simulink model "tank2_update"  (R2014a)
settings: Solver=ode1  StartTime=0.0  StopTime=inf  FixedStep=delta_t  RelTol=1e-3
PreLoadFcn:
  | model_prediction_init
undefined symbols (not defined in the file or in its folder): C_plant, delta_t, tank_area
settings Model: CovSFcnEnable=on  BufferReuse=off  Creator=Z133214  LastModifiedBy=yoshi12
settings DataIOCC: SignalLoggingSaveFormat=ModelDataLogs
settings OptimizationCC: BlockReduction=off  BooleanDataType=off  ConditionallyExecuteInputs=off  OptimizeBlockIOStorage=off  BufferReuse=off  GlobalBufferReuse=off  ExpressionFolding=off  ExpressionDepthLimit=2147483647  LocalBlockOutputs=off  OptimizeModelRefInitCode=on  LifeSpan=Inf  SimCompilerOptimization=off
settings DebuggingCC: UnderspecifiedInitializationDetection=Classic  FcnCallInpInsideContextMsg=UseLocalSettings  FrameProcessingCompatibilityMsg=error  StateNameClashWarn=warning
settings RTWCC: SystemTargetFile=ert.tlc  GenCodeOnly=on  TemplateMakefile=ert_default_tmf  Description=Real-Time Workshop Embedded Coder  RTWCompilerOptimization=off
settings CodeAppCC: IgnoreCustomStorageClasses=off  CustomSymbolStrType=$N$R$M  InternalIdentifier=Classic
settings ERTTargetCC: ParMdlRefBuildCompliant=on  CompOptLevelCompliant=on  ConcurrentExecutionCompliant=on  ERTFirstTimeCompliant=on  ModelStepFunctionPrototypeControlCompliant=on  CPPClassGenCompliant=on  InlinedParameterPlacement=Hierarchical  ERTCustomFileTemplate=example_file_process.tlc

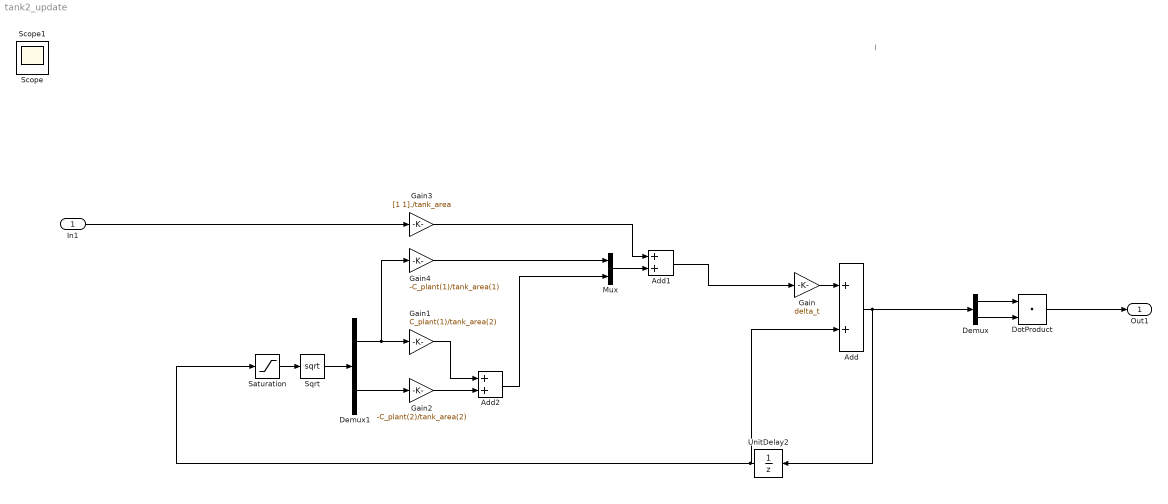
== system tank2_update ==
  note: l
  In1 : Inport
  Add : Sum
  Add1 : Sum
  Add2 : Sum
  Demux : Demux  Outputs=2
  Demux1 : Demux  Outputs=2
  DotProduct : DotProduct  InputSameDT=on  OutDataTypeStr=Inherit: Inherit via internal rule
  Gain : Gain  Gain=delta_t
  Gain1 : Gain  Gain=C_plant(1)/tank_area(2)
  Gain2 : Gain  Gain=-C_plant(2)/tank_area(2)
  Gain3 : Gain  Gain=[1 1]./tank_area
  Gain4 : Gain  Gain=-C_plant(1)/tank_area(1)
  Mux : Mux  Inputs=2
  Saturation : Saturate  UpperLimit=inf  LowerLimit=0
  Sqrt : Sqrt  SaturateOnIntegerOverflow=on
  UnitDelay2 : UnitDelay  InitialCondition=[0.01;0.01]  SampleTime=-1
  Out1 : Outport
  Scope : Scope  NumInputPorts=2
      settings: TimeRange=5  YMin=0~0  YMax=175~4  MaxDataPoints=7500
  Scope1 : Scope
      settings: MaxDataPoints=7500
  wires:
  DotProduct/1 -> Out1/1
  UnitDelay2/1 -> Add/2, Saturation/1
  Saturation/1 -> Sqrt/1
  In1/1 -> Gain3/1
  Mux/1 -> Add1/2
  Gain3/1 -> Add1/1
  Add2/1 -> Mux/2
  Gain4/1 -> Mux/1
  Gain2/1 -> Add2/2
  Gain1/1 -> Add2/1
  Demux1/2 -> Gain2/1
  Demux1/1 -> Gain1/1, Gain4/1
  Sqrt/1 -> Demux1/1
  Demux/2 -> DotProduct/2
  Demux/1 -> DotProduct/1
  Add1/1 -> Gain/1
  Gain/1 -> Add/1
  Add/1 -> Demux/1, UnitDelay2/1
